simulink model "Lift_system"  (R2020b)
settings: Solver=VariableStepAuto  StartTime=0.0  StopTime=10.0  RelTol=1e-3
settings Model: Creator=shubham sharma  LastModifiedBy=shubham sharma

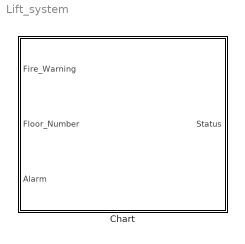
== system Lift_system ==
  Chart : Stateflow chart  TreatAsAtomicUnit=on

== stateflow chart Lift_system/Chart ==
  state Lift_Functionality [parallel]
    en: Status=0;
    settings: executionOrder=1
    note: HISTORY will remember the no. of floor where lift will be at.
    state Lift_On
      (history)
      state Ground_Floor
        en: Status=1;
        during: Floor_Number=0;
        UP_DOWN(Floor_Number);
        exit: Status=0;
      state First_Floor
        en: Status=1;
        during: Floor_Number=1;
        UP_DOWN(Floor_Number);
        exit: Status=0;
      state Second_Floor
        en: Status=1;
        during: Floor_Number=2;
        UP_DOWN(Floor_Number);
        exit: Status=0;
        after(1,sec);
      state Third_Floor
        en: Status=1;
        during: Floor_Number=3;
        UP_DOWN(Floor_Number);
        exit: Status=0;
        after(1,sec);
      state Fourth_Floor
        en: Status=1
        during: Floor_Number=4;
        UP_DOWN(Floor_Number);
        exit: Status=0;
      state Fifth_Floor
        en: Status=1;
        during: Floor_Number=5;
        UP_DOWN(Floor_Number);
        exit: Status=0;
      (default) -> Ground_Floor
      Ground_Floor -> First_Floor : UP
      First_Floor -> Ground_Floor [order 2] : DOWN
      First_Floor -> Second_Floor [order 1] : UP
      Second_Floor -> First_Floor [order 2] : DOWN
      Second_Floor -> Third_Floor [order 1] : UP
      Third_Floor -> Second_Floor [order 2] : DOWN
      Third_Floor -> Fourth_Floor [order 1] : UP
      Fourth_Floor -> Third_Floor [order 1] : DOWN
      Fourth_Floor -> Fifth_Floor [order 2] : UP
      Fifth_Floor -> Fourth_Floor : DOWN
    note: Fire warning when will change to 1 Lift's status bar will show 0.
    state Lift_Off
      en:
      Status=0;
    (default) -> Lift_On
    Lift_On -> Lift_Off : [Fire_Warning==1]
    Lift_Off -> Lift_On : [Fire_Warning==0]
  state y = UP_DOWN(Direction) [function]
    (default) -> (junction 115)
    (junction 115) -> (junction 112) [order 3] : [Select_The_Floor<Direction]{
        | send(DOWN);
        | disp('LiftMovingDown');}
    (junction 115) -> (junction 117) [order 1] : [Select_The_Floor>Direction]{
        | send(UP);
        | disp('LiftMovingUp');}
    (junction 115) -> (junction 118) [order 2] : [Select_The_Floor==Floor_Number]{
        | disp('CurrentFloor');}
    (junction 112) -> (junction 116)
    (junction 117) -> (junction 119)
    (junction 116) -> (junction 118)
    (junction 119) -> (junction 118)
    (junction 118) -> (junction 121)
  data: Direction function_input; y function_output; Fire_Warning input; Floor_Number input; Status output; Alarm input
  events: UP local FUNCTION_CALL_EVENT; DOWN local FUNCTION_CALL_EVENT; off local FUNCTION_CALL_EVENT; on local FUNCTION_CALL_EVENT
